simulink subsystem "altimeter"  (R2024b)
settings: Solver=VariableStepAuto  StartTime=0.0  StopTime=10.0  RelTol=1e-3
undefined symbols (not defined in the file or in its folder): BARO_RMSN, GROUND_LEVEL, observer_rate
libraries: simulink x1, aerolibatmos2 x1
settings Model: Creator=yevge  LastModifiedBy=yevge

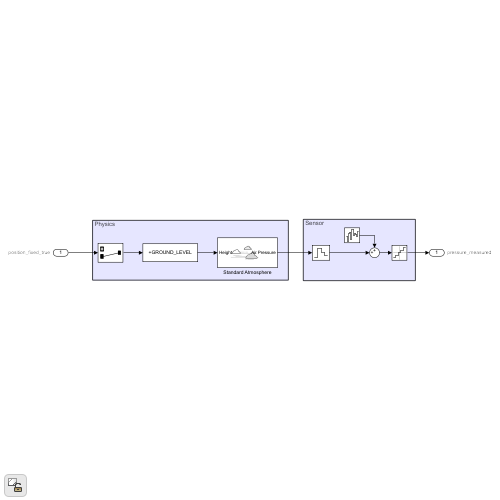
[thumbnail: Simulink's stored preview of the top-level diagram]
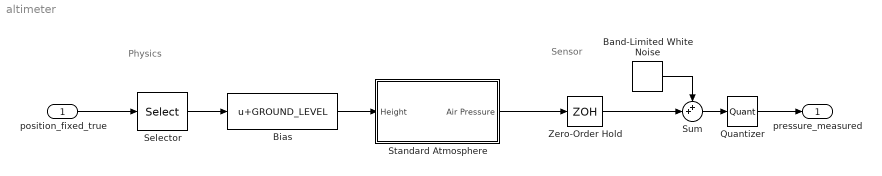
== system altimeter ==
  note: Sensor
  note: Physics
  position_fixed_true : Inport  Unit=m  PortDimensions=[2 1]
  Band-Limited White Noise : simulink/Sources/Band-Limited White Noise  Cov=BARO_RMSN^2/observer_rate  Ts=1/observer_rate  seed=[23341]
  Bias : Bias  Bias=GROUND_LEVEL  SaturateOnIntegerOverflow=off
  Quantizer : Quantizer  QuantizationInterval=BARO_QUANT
  Selector : Selector  InputPortWidth=2  IndexOptions=Index vector (dialog)  Indices=2  OutputSizes=1
  Standard Atmosphere : Subsystem
      mask Display:
      | block_icon("ISA Atmosphere Model")
      | 
      | % text(0.5 , 0.3, "ISA Pressure", ...
      | %     HorizontalAlignment="center", VerticalAlignment="middle")
      | % disp("\n\n\nISA Pressure");
  Sum : Sum  Inputs=++|
  Zero-Order Hold : ZeroOrderHold  SampleTime=1/observer_rate
  pressure_measured : Outport  Unit=Pa  PortDimensions=1  SampleTime=1/observer_rate
  wires:
  position_fixed_true/1 -> Selector/1
  Selector/1 -> Bias/1
  Quantizer/1 -> pressure_measured/1
  Bias/1 -> Standard Atmosphere/1(Height)
  Standard Atmosphere/1(Air Pressure) -> Zero-Order Hold/1
  Zero-Order Hold/1 -> Sum/2
  Sum/1 -> Quantizer/1
  Band-Limited White Noise/1 -> Sum/1

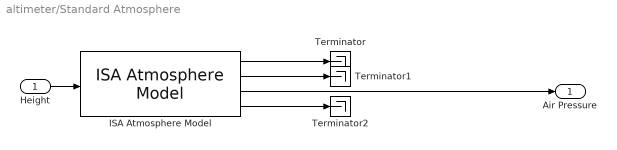
== system altimeter/Standard Atmosphere ==
  Height : Inport
  ISA Atmosphere Model : aerolibatmos2/ISA Atmosphere Model  useExtended=off  action=Warning  custom=off  viscosityOut=off  g=9.80665  gamma=1.4  R=287.0531  L=0.0065  h_trop=11000  h_strat=20000  rho0=1.225  P0=101325  T0=288.15  h0=0  S=110.4  Tref=273.15  muref=1.716e-5
  Terminator : Terminator
  Terminator1 : Terminator
  Terminator2 : Terminator
  Air Pressure : Outport
  wires:
  Height/1 -> ISA Atmosphere Model/1
  ISA Atmosphere Model/4 -> Terminator2/1
  ISA Atmosphere Model/2 -> Terminator1/1
  ISA Atmosphere Model/3 -> Air Pressure/1
  ISA Atmosphere Model/1 -> Terminator/1
